simulink model "parallel_prediction_and_cost_function_6phase"  (R2022a)
settings: Solver=FixedStepDiscrete  StartTime=0.0  StopTime=10.0  RelTol=1e-3
undefined symbols (not defined in the file or in its folder): f_c, L_d, L_q, L_x, L_y, p, psi_pm, R_ph
libraries: hdlsllib x5
(part 2 of 3)

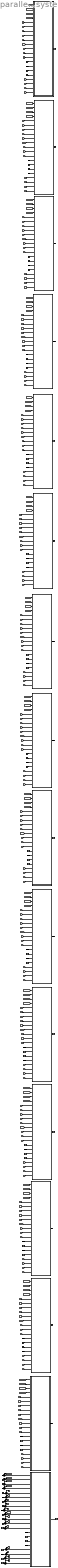
== system parallel_prediction_and_cost_function_6phase/Prediction_and_cost_function/Subsystem ==
  d_phase_voltage_per_switching_state : Inport
  q_phase_voltage_per_switching_state : Inport  Port=2
  x_phase_voltage_per_switching_state : Inport  Port=3
  y_phase_voltage_per_switching_state : Inport  Port=4
  d_phase_voltage_per_switching_state1 : Inport  Port=5
  q_phase_voltage_per_switching_state1 : Inport  Port=6
  x_phase_voltage_per_switching_state1 : Inport  Port=7
  y_phase_voltage_per_switching_state1 : Inport  Port=8
  d_phase_voltage_per_switching_state2 : Inport  Port=9
  q_phase_voltage_per_switching_state2 : Inport  Port=10
  x_phase_voltage_per_switching_state2 : Inport  Port=11
  y_phase_voltage_per_switching_state2 : Inport  Port=12
  d_phase_voltage_per_switching_state3 : Inport  Port=13
  q_phase_voltage_per_switching_state3 : Inport  Port=14
  x_phase_voltage_per_switching_state3 : Inport  Port=15
  y_phase_voltage_per_switching_state3 : Inport  Port=16
  d_phase_voltage_per_switching_state4 : Inport  Port=17
  q_phase_voltage_per_switching_state4 : Inport  Port=18
  x_phase_voltage_per_switching_state4 : Inport  Port=19
  y_phase_voltage_per_switching_state4 : Inport  Port=20
  d_phase_voltage_per_switching_state5 : Inport  Port=21
  q_phase_voltage_per_switching_state5 : Inport  Port=22
  x_phase_voltage_per_switching_state5 : Inport  Port=23
  y_phase_voltage_per_switching_state5 : Inport  Port=24
  d_phase_voltage_per_switching_state6 : Inport  Port=25
  q_phase_voltage_per_switching_state6 : Inport  Port=26
  x_phase_voltage_per_switching_state6 : Inport  Port=27
  y_phase_voltage_per_switching_state6 : Inport  Port=28
  d_phase_voltage_per_switching_state7 : Inport  Port=29
  q_phase_voltage_per_switching_state7 : Inport  Port=30
  x_phase_voltage_per_switching_state7 : Inport  Port=31
  y_phase_voltage_per_switching_state7 : Inport  Port=32
  d_phase_voltage_per_switching_state8 : Inport  Port=33
  q_phase_voltage_per_switching_state8 : Inport  Port=34
  x_phase_voltage_per_switching_state8 : Inport  Port=35
  y_phase_voltage_per_switching_state8 : Inport  Port=36
  d_phase_voltage_per_switching_state9 : Inport  Port=37
  q_phase_voltage_per_switching_state9 : Inport  Port=38
  x_phase_voltage_per_switching_state9 : Inport  Port=39
  y_phase_voltage_per_switching_state9 : Inport  Port=40
  d_phase_voltage_per_switching_state10 : Inport  Port=41
  q_phase_voltage_per_switching_state10 : Inport  Port=42
  x_phase_voltage_per_switching_state10 : Inport  Port=43
  y_phase_voltage_per_switching_state10 : Inport  Port=44
  d_phase_voltage_per_switching_state11 : Inport  Port=45
  q_phase_voltage_per_switching_state11 : Inport  Port=46
  x_phase_voltage_per_switching_state11 : Inport  Port=47
  y_phase_voltage_per_switching_state11 : Inport  Port=48
  d_phase_voltage_per_switching_state12 : Inport  Port=49
  q_phase_voltage_per_switching_state12 : Inport  Port=50
  x_phase_voltage_per_switching_state12 : Inport  Port=51
  y_phase_voltage_per_switching_state12 : Inport  Port=52
  d_phase_voltage_per_switching_state13 : Inport  Port=53
  q_phase_voltage_per_switching_state13 : Inport  Port=54
  x_phase_voltage_per_switching_state13 : Inport  Port=55
  y_phase_voltage_per_switching_state13 : Inport  Port=56
  d_phase_voltage_per_switching_state14 : Inport  Port=57
  q_phase_voltage_per_switching_state14 : Inport  Port=58
  x_phase_voltage_per_switching_state14 : Inport  Port=59
  y_phase_voltage_per_switching_state14 : Inport  Port=60
  SampleTime_div_Ld15 : Inport  Port=61
  SampleTime_div_Lq15 : Inport  Port=62
  SampleTime_div_Lx15 : Inport  Port=63
  SampleTime_div_Ly15 : Inport  Port=64
  id_k_16 : Inport  Port=65
  iq_k_16 : Inport  Port=66
  ix_k_16 : Inport  Port=67
  iy_k_16 : Inport  Port=68
  Rs15 : Inport  Port=69
  omega_el15 : Inport  Port=70
  Lq15 : Inport  Port=71
  Ld15 : Inport  Port=72
  psiPM15 : Inport  Port=73
  d_phase_voltage_per_switching_state15 : Inport  Port=74
  q_phase_voltage_per_switching_state15 : Inport  Port=75
  x_phase_voltage_per_switching_state15 : Inport  Port=76
  y_phase_voltage_per_switching_state15 : Inport  Port=77
  id_ref15 : Inport  Port=78
  iq_ref15 : Inport  Port=79
  ix_ref15 : Inport  Port=80
  iy_ref15 : Inport  Port=81
  MATLAB Function : MATLAB Function  TreatAsAtomicUnit=on
  MATLAB Function1 : MATLAB Function  TreatAsAtomicUnit=on
  MATLAB Function10 : MATLAB Function  TreatAsAtomicUnit=on
  MATLAB Function11 : MATLAB Function  TreatAsAtomicUnit=on
  MATLAB Function12 : MATLAB Function  TreatAsAtomicUnit=on
  MATLAB Function13 : MATLAB Function  TreatAsAtomicUnit=on
  MATLAB Function14 : MATLAB Function  TreatAsAtomicUnit=on
  MATLAB Function15 : MATLAB Function  TreatAsAtomicUnit=on
  MATLAB Function2 : MATLAB Function  TreatAsAtomicUnit=on
  MATLAB Function3 : MATLAB Function  TreatAsAtomicUnit=on
  MATLAB Function4 : MATLAB Function  TreatAsAtomicUnit=on
  MATLAB Function5 : MATLAB Function  TreatAsAtomicUnit=on
  MATLAB Function6 : MATLAB Function  TreatAsAtomicUnit=on
  MATLAB Function7 : MATLAB Function  TreatAsAtomicUnit=on
  MATLAB Function8 : MATLAB Function  TreatAsAtomicUnit=on
  MATLAB Function9 : MATLAB Function  TreatAsAtomicUnit=on
  J : Outport
  J1 : Outport  Port=2
  J2 : Outport  Port=3
  J3 : Outport  Port=4
  J4 : Outport  Port=5
  J5 : Outport  Port=6
  J6 : Outport  Port=7
  J7 : Outport  Port=8
  J8 : Outport  Port=9
  J9 : Outport  Port=10
  J10 : Outport  Port=11
  J11 : Outport  Port=12
  J12 : Outport  Port=13
  J13 : Outport  Port=14
  J14 : Outport  Port=15
  J15 : Outport  Port=16
  wires:
  d_phase_voltage_per_switching_state13/1 -> MATLAB Function2/14(d_phase_voltage_per_switching_state)
  q_phase_voltage_per_switching_state1/1 -> MATLAB Function14/15(q_phase_voltage_per_switching_state)
  [SampleTime_div_Ld] -> MATLAB Function15/1(SampleTime_div_Ld)
  x_phase_voltage_per_switching_state12/1 -> MATLAB Function3/16(x_phase_voltage_per_switching_state)
  [SampleTime_div_Lx] -> MATLAB Function10/3(SampleTime_div_Lx)
  SampleTime_div_Ly15/1 -> [SampleTime_div_Ly], MATLAB Function/4(SampleTime_div_Ly)
  iq_k_16/1 -> [iq_k], MATLAB Function/6(iq_k_1)
  Rs15/1 -> [Rs], MATLAB Function/9(Rs)
  iy_k_16/1 -> [iy_k], MATLAB Function/8(iy_k_1)
  MATLAB Function/1(J) -> J15/1
  y_phase_voltage_per_switching_state/1 -> MATLAB Function15/17(y_phase_voltage_per_switching_state)
  Lq15/1 -> [Lq], MATLAB Function/11(Lq)
  x_phase_voltage_per_switching_state15/1 -> MATLAB Function/16(x_phase_voltage_per_switching_state)
  MATLAB Function11/1(J) -> J4/1
  SampleTime_div_Lq15/1 -> [SampleTime_div_Lq], MATLAB Function/2(SampleTime_div_Lq)
  MATLAB Function4/1(J) -> J11/1
  y_phase_voltage_per_switching_state2/1 -> MATLAB Function13/17(y_phase_voltage_per_switching_state)
  d_phase_voltage_per_switching_state1/1 -> MATLAB Function14/14(d_phase_voltage_per_switching_state)
  iq_ref15/1 -> [iq_ref], MATLAB Function/19(iq_ref)
  SampleTime_div_Lx15/1 -> [SampleTime_div_Lx], MATLAB Function/3(SampleTime_div_Lx)
  d_phase_voltage_per_switching_state15/1 -> MATLAB Function/14(d_phase_voltage_per_switching_state)
  x_phase_voltage_per_switching_state1/1 -> MATLAB Function14/16(x_phase_voltage_per_switching_state)
  y_phase_voltage_per_switching_state7/1 -> MATLAB Function8/17(y_phase_voltage_per_switching_state)
  iy_ref15/1 -> [iy_ref], MATLAB Function/21(iy_ref)
  id_ref15/1 -> [id_ref], MATLAB Function/18(id_ref)
  id_k_16/1 -> [id_k], MATLAB Function/5(id_k_1)
  omega_el15/1 -> [omega_el], MATLAB Function/10(omega_el)
  ix_k_16/1 -> [ix_k], MATLAB Function/7(ix_k_1)
  psiPM15/1 -> [psiPM], MATLAB Function/13(psiPM)
  [iq_k] -> MATLAB Function10/6(iq_k_1)
  MATLAB Function1/1(J) -> J14/1
  ix_ref15/1 -> [ix_ref], MATLAB Function/20(ix_ref)
  d_phase_voltage_per_switching_state3/1 -> MATLAB Function12/14(d_phase_voltage_per_switching_state)
  SampleTime_div_Ld15/1 -> [SampleTime_div_Ld], MATLAB Function/1(SampleTime_div_Ld)
  d_phase_voltage_per_switching_state6/1 -> MATLAB Function9/14(d_phase_voltage_per_switching_state)
  x_phase_voltage_per_switching_state9/1 -> MATLAB Function6/16(x_phase_voltage_per_switching_state)
  d_phase_voltage_per_switching_state/1 -> MATLAB Function15/14(d_phase_voltage_per_switching_state)
  x_phase_voltage_per_switching_state3/1 -> MATLAB Function12/16(x_phase_voltage_per_switching_state)
  y_phase_voltage_per_switching_state15/1 -> MATLAB Function/17(y_phase_voltage_per_switching_state)
  d_phase_voltage_per_switching_state2/1 -> MATLAB Function13/14(d_phase_voltage_per_switching_state)
  q_phase_voltage_per_switching_state15/1 -> MATLAB Function/15(q_phase_voltage_per_switching_state)
  x_phase_voltage_per_switching_state8/1 -> MATLAB Function7/16(x_phase_voltage_per_switching_state)
  y_phase_voltage_per_switching_state9/1 -> MATLAB Function6/17(y_phase_voltage_per_switching_state)
  x_phase_voltage_per_switching_state4/1 -> MATLAB Function11/16(x_phase_voltage_per_switching_state)
  y_phase_voltage_per_switching_state1/1 -> MATLAB Function14/17(y_phase_voltage_per_switching_state)
  MATLAB Function14/1(J) -> J1/1
  MATLAB Function8/1(J) -> J7/1
  [ix_ref] -> MATLAB Function2/20(ix_ref)
  q_phase_voltage_per_switching_state2/1 -> MATLAB Function13/15(q_phase_voltage_per_switching_state)
  x_phase_voltage_per_switching_state2/1 -> MATLAB Function13/16(x_phase_voltage_per_switching_state)
  [iq_ref] -> MATLAB Function9/19(iq_ref)
  MATLAB Function13/1(J) -> J2/1
  y_phase_voltage_per_switching_state11/1 -> MATLAB Function4/17(y_phase_voltage_per_switching_state)
  [SampleTime_div_Ly] -> MATLAB Function10/4(SampleTime_div_Ly)
  y_phase_voltage_per_switching_state4/1 -> MATLAB Function11/17(y_phase_voltage_per_switching_state)
  x_phase_voltage_per_switching_state/1 -> MATLAB Function15/16(x_phase_voltage_per_switching_state)
  d_phase_voltage_per_switching_state14/1 -> MATLAB Function1/14(d_phase_voltage_per_switching_state)
  q_phase_voltage_per_switching_state9/1 -> MATLAB Function6/15(q_phase_voltage_per_switching_state)
  q_phase_voltage_per_switching_state5/1 -> MATLAB Function10/15(q_phase_voltage_per_switching_state)
  d_phase_voltage_per_switching_state10/1 -> MATLAB Function5/14(d_phase_voltage_per_switching_state)
  x_phase_voltage_per_switching_state14/1 -> MATLAB Function1/16(x_phase_voltage_per_switching_state)
  y_phase_voltage_per_switching_state14/1 -> MATLAB Function1/17(y_phase_voltage_per_switching_state)
  q_phase_voltage_per_switching_state14/1 -> MATLAB Function1/15(q_phase_voltage_per_switching_state)
  [iy_k] -> MATLAB Function10/8(iy_k_1)
  q_phase_voltage_per_switching_state11/1 -> MATLAB Function4/15(q_phase_voltage_per_switching_state)
  x_phase_voltage_per_switching_state11/1 -> MATLAB Function4/16(x_phase_voltage_per_switching_state)
  d_phase_voltage_per_switching_state11/1 -> MATLAB Function4/14(d_phase_voltage_per_switching_state)
  MATLAB Function2/1(J) -> J13/1
  y_phase_voltage_per_switching_state12/1 -> MATLAB Function3/17(y_phase_voltage_per_switching_state)
  x_phase_voltage_per_switching_state13/1 -> MATLAB Function2/16(x_phase_voltage_per_switching_state)
  [SampleTime_div_Ld] -> MATLAB Function12/1(SampleTime_div_Ld)
  [id_ref] -> MATLAB Function2/18(id_ref)
  d_phase_voltage_per_switching_state9/1 -> MATLAB Function6/14(d_phase_voltage_per_switching_state)
  MATLAB Function6/1(J) -> J9/1
  d_phase_voltage_per_switching_state7/1 -> MATLAB Function8/14(d_phase_voltage_per_switching_state)
  d_phase_voltage_per_switching_state4/1 -> MATLAB Function11/14(d_phase_voltage_per_switching_state)
  q_phase_voltage_per_switching_state4/1 -> MATLAB Function11/15(q_phase_voltage_per_switching_state)
  q_phase_voltage_per_switching_state12/1 -> MATLAB Function3/15(q_phase_voltage_per_switching_state)
  [iy_ref] -> MATLAB Function2/21(iy_ref)
  d_phase_voltage_per_switching_state8/1 -> MATLAB Function7/14(d_phase_voltage_per_switching_state)
  x_phase_voltage_per_switching_state5/1 -> MATLAB Function10/16(x_phase_voltage_per_switching_state)
  d_phase_voltage_per_switching_state12/1 -> MATLAB Function3/14(d_phase_voltage_per_switching_state)
  MATLAB Function3/1(J) -> J12/1
  [SampleTime_div_Lx] -> MATLAB Function15/3(SampleTime_div_Lx)
  [SampleTime_div_Ly] -> MATLAB Function15/4(SampleTime_div_Ly)
  [SampleTime_div_Lq] -> MATLAB Function15/2(SampleTime_div_Lq)
  [SampleTime_div_Ld] -> MATLAB Function10/1(SampleTime_div_Ld)
  [SampleTime_div_Lx] -> MATLAB Function12/3(SampleTime_div_Lx)
  [SampleTime_div_Lq] -> MATLAB Function10/2(SampleTime_div_Lq)
  x_phase_voltage_per_switching_state7/1 -> MATLAB Function8/16(x_phase_voltage_per_switching_state)
  q_phase_voltage_per_switching_state/1 -> MATLAB Function15/15(q_phase_voltage_per_switching_state)
  [SampleTime_div_Lq] -> MATLAB Function12/2(SampleTime_div_Lq)
  MATLAB Function15/1(J) -> J/1
  [id_k] -> MATLAB Function10/5(id_k_1)
  [ix_k] -> MATLAB Function10/7(ix_k_1)
  d_phase_voltage_per_switching_state5/1 -> MATLAB Function10/14(d_phase_voltage_per_switching_state)
  q_phase_voltage_per_switching_state13/1 -> MATLAB Function2/15(q_phase_voltage_per_switching_state)
  MATLAB Function10/1(J) -> J5/1
  y_phase_voltage_per_switching_state5/1 -> MATLAB Function10/17(y_phase_voltage_per_switching_state)
  MATLAB Function5/1(J) -> J10/1
  q_phase_voltage_per_switching_state6/1 -> MATLAB Function9/15(q_phase_voltage_per_switching_state)
  y_phase_voltage_per_switching_state6/1 -> MATLAB Function9/17(y_phase_voltage_per_switching_state)
  [ix_ref] -> MATLAB Function9/20(ix_ref)
  [id_ref] -> MATLAB Function9/18(id_ref)
  x_phase_voltage_per_switching_state6/1 -> MATLAB Function9/16(x_phase_voltage_per_switching_state)
  MATLAB Function9/1(J) -> J6/1
  [iy_ref] -> MATLAB Function9/21(iy_ref)
  y_phase_voltage_per_switching_state8/1 -> MATLAB Function7/17(y_phase_voltage_per_switching_state)
  MATLAB Function12/1(J) -> J3/1
  q_phase_voltage_per_switching_state8/1 -> MATLAB Function7/15(q_phase_voltage_per_switching_state)
  y_phase_voltage_per_switching_state13/1 -> MATLAB Function2/17(y_phase_voltage_per_switching_state)
  MATLAB Function7/1(J) -> J8/1
  q_phase_voltage_per_switching_state7/1 -> MATLAB Function8/15(q_phase_voltage_per_switching_state)
  [iq_ref] -> MATLAB Function2/19(iq_ref)
  [SampleTime_div_Ly] -> MATLAB Function12/4(SampleTime_div_Ly)
  x_phase_voltage_per_switching_state10/1 -> MATLAB Function5/16(x_phase_voltage_per_switching_state)
  q_phase_voltage_per_switching_state10/1 -> MATLAB Function5/15(q_phase_voltage_per_switching_state)
  y_phase_voltage_per_switching_state10/1 -> MATLAB Function5/17(y_phase_voltage_per_switching_state)
  y_phase_voltage_per_switching_state3/1 -> MATLAB Function12/17(y_phase_voltage_per_switching_state)
  q_phase_voltage_per_switching_state3/1 -> MATLAB Function12/15(q_phase_voltage_per_switching_state)
  [SampleTime_div_Ld] -> MATLAB Function1/1(SampleTime_div_Ld)
  [SampleTime_div_Ld] -> MATLAB Function2/1(SampleTime_div_Ld)
  [SampleTime_div_Ld] -> MATLAB Function3/1(SampleTime_div_Ld)
  [SampleTime_div_Ld] -> MATLAB Function4/1(SampleTime_div_Ld)
  [SampleTime_div_Ld] -> MATLAB Function6/1(SampleTime_div_Ld)
  [SampleTime_div_Ld] -> MATLAB Function5/1(SampleTime_div_Ld)
  [SampleTime_div_Ld] -> MATLAB Function7/1(SampleTime_div_Ld)
  [SampleTime_div_Ld] -> MATLAB Function8/1(SampleTime_div_Ld)
  [SampleTime_div_Ld] -> MATLAB Function9/1(SampleTime_div_Ld)
  [SampleTime_div_Ld] -> MATLAB Function11/1(SampleTime_div_Ld)
  [SampleTime_div_Ld] -> MATLAB Function13/1(SampleTime_div_Ld)
  [SampleTime_div_Ld] -> MATLAB Function14/1(SampleTime_div_Ld)
  [SampleTime_div_Lq] -> MATLAB Function1/2(SampleTime_div_Lq)
  [SampleTime_div_Lq] -> MATLAB Function2/2(SampleTime_div_Lq)
  [SampleTime_div_Lq] -> MATLAB Function3/2(SampleTime_div_Lq)
  [SampleTime_div_Lq] -> MATLAB Function4/2(SampleTime_div_Lq)
  [SampleTime_div_Lq] -> MATLAB Function5/2(SampleTime_div_Lq)
  [SampleTime_div_Lq] -> MATLAB Function6/2(SampleTime_div_Lq)
  [SampleTime_div_Lq] -> MATLAB Function7/2(SampleTime_div_Lq)
  [SampleTime_div_Lq] -> MATLAB Function8/2(SampleTime_div_Lq)
  [SampleTime_div_Lq] -> MATLAB Function9/2(SampleTime_div_Lq)
  [SampleTime_div_Lq] -> MATLAB Function11/2(SampleTime_div_Lq)
  [SampleTime_div_Lq] -> MATLAB Function13/2(SampleTime_div_Lq)
  [SampleTime_div_Lq] -> MATLAB Function14/2(SampleTime_div_Lq)
  [SampleTime_div_Lx] -> MATLAB Function1/3(SampleTime_div_Lx)
  [SampleTime_div_Lx] -> MATLAB Function2/3(SampleTime_div_Lx)
  [SampleTime_div_Lx] -> MATLAB Function3/3(SampleTime_div_Lx)
  [SampleTime_div_Lx] -> MATLAB Function4/3(SampleTime_div_Lx)
  [SampleTime_div_Lx] -> MATLAB Function5/3(SampleTime_div_Lx)
  [SampleTime_div_Lx] -> MATLAB Function6/3(SampleTime_div_Lx)
  [SampleTime_div_Lx] -> MATLAB Function7/3(SampleTime_div_Lx)
  [SampleTime_div_Lx] -> MATLAB Function8/3(SampleTime_div_Lx)
  [SampleTime_div_Lx] -> MATLAB Function9/3(SampleTime_div_Lx)
  [SampleTime_div_Lx] -> MATLAB Function11/3(SampleTime_div_Lx)
  [SampleTime_div_Lx] -> MATLAB Function13/3(SampleTime_div_Lx)
  [SampleTime_div_Lx] -> MATLAB Function14/3(SampleTime_div_Lx)
  [SampleTime_div_Ly] -> MATLAB Function1/4(SampleTime_div_Ly)
  [SampleTime_div_Ly] -> MATLAB Function2/4(SampleTime_div_Ly)
  [SampleTime_div_Ly] -> MATLAB Function3/4(SampleTime_div_Ly)
  [SampleTime_div_Ly] -> MATLAB Function4/4(SampleTime_div_Ly)
  [SampleTime_div_Ly] -> MATLAB Function5/4(SampleTime_div_Ly)
  [SampleTime_div_Ly] -> MATLAB Function6/4(SampleTime_div_Ly)
  [SampleTime_div_Ly] -> MATLAB Function7/4(SampleTime_div_Ly)
  [SampleTime_div_Ly] -> MATLAB Function8/4(SampleTime_div_Ly)
  [SampleTime_div_Ly] -> MATLAB Function9/4(SampleTime_div_Ly)
  [SampleTime_div_Ly] -> MATLAB Function11/4(SampleTime_div_Ly)
  [SampleTime_div_Ly] -> MATLAB Function13/4(SampleTime_div_Ly)
  [SampleTime_div_Ly] -> MATLAB Function14/4(SampleTime_div_Ly)
  [id_k] -> MATLAB Function1/5(id_k_1)
  [iq_k] -> MATLAB Function1/6(iq_k_1)
  [ix_k] -> MATLAB Function1/7(ix_k_1)
  [iy_k] -> MATLAB Function1/8(iy_k_1)
  [Rs] -> MATLAB Function1/9(Rs)
  [omega_el] -> MATLAB Function1/10(omega_el)
  [Lq] -> MATLAB Function1/11(Lq)
  Ld15/1 -> [Ld], MATLAB Function/12(Ld)
  [Ld] -> MATLAB Function1/12(Ld)
  [psiPM] -> MATLAB Function1/13(psiPM)
  [id_ref] -> MATLAB Function1/18(id_ref)
  [iq_ref] -> MATLAB Function1/19(iq_ref)
  [ix_ref] -> MATLAB Function1/20(ix_ref)
  [iy_ref] -> MATLAB Function1/21(iy_ref)
  [Ld] -> MATLAB Function2/12(Ld)
  [omega_el] -> MATLAB Function2/10(omega_el)
  [iy_k] -> MATLAB Function2/8(iy_k_1)
  [Lq] -> MATLAB Function2/11(Lq)
  [psiPM] -> MATLAB Function2/13(psiPM)
  [iq_k] -> MATLAB Function2/6(iq_k_1)
  [id_k] -> MATLAB Function2/5(id_k_1)
  [ix_k] -> MATLAB Function2/7(ix_k_1)
  [Rs] -> MATLAB Function2/9(Rs)
  [Ld] -> MATLAB Function3/12(Ld)
  [omega_el] -> MATLAB Function3/10(omega_el)
  [iy_k] -> MATLAB Function3/8(iy_k_1)
  [Lq] -> MATLAB Function3/11(Lq)
  [psiPM] -> MATLAB Function3/13(psiPM)
  [iq_ref] -> MATLAB Function3/19(iq_ref)
  [iq_k] -> MATLAB Function3/6(iq_k_1)
  [id_k] -> MATLAB Function3/5(id_k_1)
  [iy_ref] -> MATLAB Function3/21(iy_ref)
  [ix_k] -> MATLAB Function3/7(ix_k_1)
  [Rs] -> MATLAB Function3/9(Rs)
  [id_ref] -> MATLAB Function3/18(id_ref)
  [ix_ref] -> MATLAB Function3/20(ix_ref)
  [Ld] -> MATLAB Function4/12(Ld)
  [omega_el] -> MATLAB Function4/10(omega_el)
  [iy_k] -> MATLAB Function4/8(iy_k_1)
  [Lq] -> MATLAB Function4/11(Lq)
  [psiPM] -> MATLAB Function4/13(psiPM)
  [iq_ref] -> MATLAB Function4/19(iq_ref)
  [iq_k] -> MATLAB Function4/6(iq_k_1)
  [id_k] -> MATLAB Function4/5(id_k_1)
  [iy_ref] -> MATLAB Function4/21(iy_ref)
  [ix_k] -> MATLAB Function4/7(ix_k_1)
  [Rs] -> MATLAB Function4/9(Rs)
  [id_ref] -> MATLAB Function4/18(id_ref)
  [ix_ref] -> MATLAB Function4/20(ix_ref)
  [Ld] -> MATLAB Function5/12(Ld)
  [omega_el] -> MATLAB Function5/10(omega_el)
  [iy_k] -> MATLAB Function5/8(iy_k_1)
  [Lq] -> MATLAB Function5/11(Lq)
  [psiPM] -> MATLAB Function5/13(psiPM)
  [iq_ref] -> MATLAB Function5/19(iq_ref)
  [iq_k] -> MATLAB Function5/6(iq_k_1)
  [id_k] -> MATLAB Function5/5(id_k_1)
  [iy_ref] -> MATLAB Function5/21(iy_ref)
  [ix_k] -> MATLAB Function5/7(ix_k_1)
  [Rs] -> MATLAB Function5/9(Rs)
  [id_ref] -> MATLAB Function5/18(id_ref)
  [ix_ref] -> MATLAB Function5/20(ix_ref)
  [Ld] -> MATLAB Function6/12(Ld)
  [omega_el] -> MATLAB Function6/10(omega_el)
  [iy_k] -> MATLAB Function6/8(iy_k_1)
  [Lq] -> MATLAB Function6/11(Lq)
  [psiPM] -> MATLAB Function6/13(psiPM)
  [iq_ref] -> MATLAB Function6/19(iq_ref)
  [iq_k] -> MATLAB Function6/6(iq_k_1)
  [id_k] -> MATLAB Function6/5(id_k_1)
  [iy_ref] -> MATLAB Function6/21(iy_ref)
  [ix_k] -> MATLAB Function6/7(ix_k_1)
  [Rs] -> MATLAB Function6/9(Rs)
  [id_ref] -> MATLAB Function6/18(id_ref)
  [ix_ref] -> MATLAB Function6/20(ix_ref)
  [Ld] -> MATLAB Function7/12(Ld)
  [omega_el] -> MATLAB Function7/10(omega_el)
  [iy_k] -> MATLAB Function7/8(iy_k_1)
  [Lq] -> MATLAB Function7/11(Lq)
  [psiPM] -> MATLAB Function7/13(psiPM)
  [iq_ref] -> MATLAB Function7/19(iq_ref)
  [iq_k] -> MATLAB Function7/6(iq_k_1)
  [id_k] -> MATLAB Function7/5(id_k_1)
  [iy_ref] -> MATLAB Function7/21(iy_ref)
  [ix_k] -> MATLAB Function7/7(ix_k_1)
  [Rs] -> MATLAB Function7/9(Rs)
  [id_ref] -> MATLAB Function7/18(id_ref)
  [ix_ref] -> MATLAB Function7/20(ix_ref)
  [Ld] -> MATLAB Function8/12(Ld)
  [omega_el] -> MATLAB Function8/10(omega_el)
  [iy_k] -> MATLAB Function8/8(iy_k_1)
  [Lq] -> MATLAB Function8/11(Lq)
  [psiPM] -> MATLAB Function8/13(psiPM)
  [iq_ref] -> MATLAB Function8/19(iq_ref)
  [iq_k] -> MATLAB Function8/6(iq_k_1)
  [id_k] -> MATLAB Function8/5(id_k_1)
  [iy_ref] -> MATLAB Function8/21(iy_ref)
  [ix_k] -> MATLAB Function8/7(ix_k_1)
  [Rs] -> MATLAB Function8/9(Rs)
  [id_ref] -> MATLAB Function8/18(id_ref)
  [ix_ref] -> MATLAB Function8/20(ix_ref)
  [Ld] -> MATLAB Function9/12(Ld)
  [omega_el] -> MATLAB Function9/10(omega_el)
  [iy_k] -> MATLAB Function9/8(iy_k_1)
  [Lq] -> MATLAB Function9/11(Lq)
  [psiPM] -> MATLAB Function9/13(psiPM)
  [iq_k] -> MATLAB Function9/6(iq_k_1)
  [id_k] -> MATLAB Function9/5(id_k_1)
  [ix_k] -> MATLAB Function9/7(ix_k_1)
  [Rs] -> MATLAB Function9/9(Rs)
  [Ld] -> MATLAB Function10/12(Ld)
  [Lq] -> MATLAB Function10/11(Lq)
  [psiPM] -> MATLAB Function10/13(psiPM)
  [iq_ref] -> MATLAB Function10/19(iq_ref)
  [iy_ref] -> MATLAB Function10/21(iy_ref)
  [id_ref] -> MATLAB Function10/18(id_ref)
  [ix_ref] -> MATLAB Function10/20(ix_ref)
  [Rs] -> MATLAB Function10/9(Rs)
  [omega_el] -> MATLAB Function10/10(omega_el)
  [Ld] -> MATLAB Function11/12(Ld)
  [omega_el] -> MATLAB Function11/10(omega_el)
  [iy_k] -> MATLAB Function11/8(iy_k_1)
  [Lq] -> MATLAB Function11/11(Lq)
  [psiPM] -> MATLAB Function11/13(psiPM)
  [iq_ref] -> MATLAB Function11/19(iq_ref)
  [iq_k] -> MATLAB Function11/6(iq_k_1)
  [id_k] -> MATLAB Function11/5(id_k_1)
  [iy_ref] -> MATLAB Function11/21(iy_ref)
  [ix_k] -> MATLAB Function11/7(ix_k_1)
  [Rs] -> MATLAB Function11/9(Rs)
  [id_ref] -> MATLAB Function11/18(id_ref)
  [ix_ref] -> MATLAB Function11/20(ix_ref)
  [Ld] -> MATLAB Function12/12(Ld)
  [omega_el] -> MATLAB Function12/10(omega_el)
  [iy_k] -> MATLAB Function12/8(iy_k_1)
  [Lq] -> MATLAB Function12/11(Lq)
  [psiPM] -> MATLAB Function12/13(psiPM)
  [iq_ref] -> MATLAB Function12/19(iq_ref)
  [iq_k] -> MATLAB Function12/6(iq_k_1)
  [id_k] -> MATLAB Function12/5(id_k_1)
  [iy_ref] -> MATLAB Function12/21(iy_ref)
  [ix_k] -> MATLAB Function12/7(ix_k_1)
  [Rs] -> MATLAB Function12/9(Rs)
  [id_ref] -> MATLAB Function12/18(id_ref)
  [ix_ref] -> MATLAB Function12/20(ix_ref)
  [Ld] -> MATLAB Function13/12(Ld)
  [omega_el] -> MATLAB Function13/10(omega_el)
  [iy_k] -> MATLAB Function13/8(iy_k_1)
  [Lq] -> MATLAB Function13/11(Lq)
  [psiPM] -> MATLAB Function13/13(psiPM)
  [iq_ref] -> MATLAB Function13/19(iq_ref)
  [iq_k] -> MATLAB Function13/6(iq_k_1)
  [id_k] -> MATLAB Function13/5(id_k_1)
  [iy_ref] -> MATLAB Function13/21(iy_ref)
  [ix_k] -> MATLAB Function13/7(ix_k_1)
  [Rs] -> MATLAB Function13/9(Rs)
  [id_ref] -> MATLAB Function13/18(id_ref)
  [ix_ref] -> MATLAB Function13/20(ix_ref)
  [Ld] -> MATLAB Function14/12(Ld)
  [omega_el] -> MATLAB Function14/10(omega_el)
  [iy_k] -> MATLAB Function14/8(iy_k_1)
  [Lq] -> MATLAB Function14/11(Lq)
  [psiPM] -> MATLAB Function14/13(psiPM)
  [iq_ref] -> MATLAB Function14/19(iq_ref)
  [iq_k] -> MATLAB Function14/6(iq_k_1)
  [id_k] -> MATLAB Function14/5(id_k_1)
  [iy_ref] -> MATLAB Function14/21(iy_ref)
  [ix_k] -> MATLAB Function14/7(ix_k_1)
  [Rs] -> MATLAB Function14/9(Rs)
  [id_ref] -> MATLAB Function14/18(id_ref)
  [ix_ref] -> MATLAB Function14/20(ix_ref)
  [Ld] -> MATLAB Function15/12(Ld)
  [omega_el] -> MATLAB Function15/10(omega_el)
  [iy_k] -> MATLAB Function15/8(iy_k_1)
  [Lq] -> MATLAB Function15/11(Lq)
  [psiPM] -> MATLAB Function15/13(psiPM)
  [iq_ref] -> MATLAB Function15/19(iq_ref)
  [iq_k] -> MATLAB Function15/6(iq_k_1)
  [id_k] -> MATLAB Function15/5(id_k_1)
  [iy_ref] -> MATLAB Function15/21(iy_ref)
  [ix_k] -> MATLAB Function15/7(ix_k_1)
  [Rs] -> MATLAB Function15/9(Rs)
  [id_ref] -> MATLAB Function15/18(id_ref)
  [ix_ref] -> MATLAB Function15/20(ix_ref)

== matlab function parallel_prediction_and_cost_function_6phase/Prediction_and_cost_function/Subsystem/MATLAB Function3 ==
  data: SampleTime_div_Ld input; J output; SampleTime_div_Lq input; SampleTime_div_Lx input; SampleTime_div_Ly input; id_k_1 input; iq_k_1 input; ix_k_1 input; iy_k_1 input; Rs input; omega_el input; Lq input; Ld input; psiPM input; d_phase_voltage_per_switching_state input; q_phase_voltage_per_switching_state input; x_phase_voltage_per_switching_state input; y_phase_voltage_per_switching_state input; id_ref input; iq_ref input; ix_ref input; iy_ref input
function J = fcn(SampleTime_div_Ld, SampleTime_div_Lq, SampleTime_div_Lx, SampleTime_div_Ly, id_k_1, iq_k_1, ix_k_1, iy_k_1, Rs, omega_el, Lq, Ld, psiPM, d_phase_voltage_per_switching_state, q_phase_voltage_per_switching_state, x_phase_voltage_per_switching_state, y_phase_voltage_per_switching_state, id_ref, iq_ref, ix_ref, iy_ref)
     
        % Prediction of the d-, q-, x-, y-currents of the 6-Phase-PMSM with the finite control set 
        id_k_2 = single(SampleTime_div_Ld*(d_phase_voltage_per_switching_state-id_k_1*Rs+omega_el*Lq*iq_k_1)+id_k_1);
        iq_k_2 = single(SampleTime_div_Lq*(q_phase_voltage_per_switching_state-iq_k_1*Rs-omega_el*(psiPM+id_k_1*Ld))+iq_k_1);
        ix_k_2 = single(SampleTime_div_Lx*(x_phase_voltage_per_switching_state-ix_k_1*Rs)+ix_k_1);
        iy_k_2 = single(SampleTime_div_Ly*(y_phase_voltage_per_switching_state-iy_k_1*Rs)+iy_k_1);
        
        % Calculation of the cost function
        J = single((id_ref-id_k_2)^2+(iq_ref-iq_k_2)^2+(ix_ref-ix_k_2)^2+(iy_ref-iy_k_2)^2);

end

== matlab function parallel_prediction_and_cost_function_6phase/Prediction_and_cost_function/Subsystem/MATLAB Function4 ==
  data: SampleTime_div_Ld input; J output; SampleTime_div_Lq input; SampleTime_div_Lx input; SampleTime_div_Ly input; id_k_1 input; iq_k_1 input; ix_k_1 input; iy_k_1 input; Rs input; omega_el input; Lq input; Ld input; psiPM input; d_phase_voltage_per_switching_state input; q_phase_voltage_per_switching_state input; x_phase_voltage_per_switching_state input; y_phase_voltage_per_switching_state input; id_ref input; iq_ref input; ix_ref input; iy_ref input
function J = fcn(SampleTime_div_Ld, SampleTime_div_Lq, SampleTime_div_Lx, SampleTime_div_Ly, id_k_1, iq_k_1, ix_k_1, iy_k_1, Rs, omega_el, Lq, Ld, psiPM, d_phase_voltage_per_switching_state, q_phase_voltage_per_switching_state, x_phase_voltage_per_switching_state, y_phase_voltage_per_switching_state, id_ref, iq_ref, ix_ref, iy_ref)
     
        % Prediction of the d-, q-, x-, y-currents of the 6-Phase-PMSM with the finite control set 
        id_k_2 = single(SampleTime_div_Ld*(d_phase_voltage_per_switching_state-id_k_1*Rs+omega_el*Lq*iq_k_1)+id_k_1);
        iq_k_2 = single(SampleTime_div_Lq*(q_phase_voltage_per_switching_state-iq_k_1*Rs-omega_el*(psiPM+id_k_1*Ld))+iq_k_1);
        ix_k_2 = single(SampleTime_div_Lx*(x_phase_voltage_per_switching_state-ix_k_1*Rs)+ix_k_1);
        iy_k_2 = single(SampleTime_div_Ly*(y_phase_voltage_per_switching_state-iy_k_1*Rs)+iy_k_1);
        
        % Calculation of the cost function
        J = single((id_ref-id_k_2)^2+(iq_ref-iq_k_2)^2+(ix_ref-ix_k_2)^2+(iy_ref-iy_k_2)^2);

end

== matlab function parallel_prediction_and_cost_function_6phase/Prediction_and_cost_function/Subsystem/MATLAB Function5 ==
  data: SampleTime_div_Ld input; J output; SampleTime_div_Lq input; SampleTime_div_Lx input; SampleTime_div_Ly input; id_k_1 input; iq_k_1 input; ix_k_1 input; iy_k_1 input; Rs input; omega_el input; Lq input; Ld input; psiPM input; d_phase_voltage_per_switching_state input; q_phase_voltage_per_switching_state input; x_phase_voltage_per_switching_state input; y_phase_voltage_per_switching_state input; id_ref input; iq_ref input; ix_ref input; iy_ref input
function J = fcn(SampleTime_div_Ld, SampleTime_div_Lq, SampleTime_div_Lx, SampleTime_div_Ly, id_k_1, iq_k_1, ix_k_1, iy_k_1, Rs, omega_el, Lq, Ld, psiPM, d_phase_voltage_per_switching_state, q_phase_voltage_per_switching_state, x_phase_voltage_per_switching_state, y_phase_voltage_per_switching_state, id_ref, iq_ref, ix_ref, iy_ref)
     
        % Prediction of the d-, q-, x-, y-currents of the 6-Phase-PMSM with the finite control set 
        id_k_2 = single(SampleTime_div_Ld*(d_phase_voltage_per_switching_state-id_k_1*Rs+omega_el*Lq*iq_k_1)+id_k_1);
        iq_k_2 = single(SampleTime_div_Lq*(q_phase_voltage_per_switching_state-iq_k_1*Rs-omega_el*(psiPM+id_k_1*Ld))+iq_k_1);
        ix_k_2 = single(SampleTime_div_Lx*(x_phase_voltage_per_switching_state-ix_k_1*Rs)+ix_k_1);
        iy_k_2 = single(SampleTime_div_Ly*(y_phase_voltage_per_switching_state-iy_k_1*Rs)+iy_k_1);
        
        % Calculation of the cost function
        J = single((id_ref-id_k_2)^2+(iq_ref-iq_k_2)^2+(ix_ref-ix_k_2)^2+(iy_ref-iy_k_2)^2);

end

== matlab function parallel_prediction_and_cost_function_6phase/Prediction_and_cost_function/Subsystem/MATLAB Function6 ==
  data: SampleTime_div_Ld input; J output; SampleTime_div_Lq input; SampleTime_div_Lx input; SampleTime_div_Ly input; id_k_1 input; iq_k_1 input; ix_k_1 input; iy_k_1 input; Rs input; omega_el input; Lq input; Ld input; psiPM input; d_phase_voltage_per_switching_state input; q_phase_voltage_per_switching_state input; x_phase_voltage_per_switching_state input; y_phase_voltage_per_switching_state input; id_ref input; iq_ref input; ix_ref input; iy_ref input
function J = fcn(SampleTime_div_Ld, SampleTime_div_Lq, SampleTime_div_Lx, SampleTime_div_Ly, id_k_1, iq_k_1, ix_k_1, iy_k_1, Rs, omega_el, Lq, Ld, psiPM, d_phase_voltage_per_switching_state, q_phase_voltage_per_switching_state, x_phase_voltage_per_switching_state, y_phase_voltage_per_switching_state, id_ref, iq_ref, ix_ref, iy_ref)
     
        % Prediction of the d-, q-, x-, y-currents of the 6-Phase-PMSM with the finite control set 
        id_k_2 = single(SampleTime_div_Ld*(d_phase_voltage_per_switching_state-id_k_1*Rs+omega_el*Lq*iq_k_1)+id_k_1);
        iq_k_2 = single(SampleTime_div_Lq*(q_phase_voltage_per_switching_state-iq_k_1*Rs-omega_el*(psiPM+id_k_1*Ld))+iq_k_1);
        ix_k_2 = single(SampleTime_div_Lx*(x_phase_voltage_per_switching_state-ix_k_1*Rs)+ix_k_1);
        iy_k_2 = single(SampleTime_div_Ly*(y_phase_voltage_per_switching_state-iy_k_1*Rs)+iy_k_1);
        
        % Calculation of the cost function
        J = single((id_ref-id_k_2)^2+(iq_ref-iq_k_2)^2+(ix_ref-ix_k_2)^2+(iy_ref-iy_k_2)^2);

end

== matlab function parallel_prediction_and_cost_function_6phase/Prediction_and_cost_function/Subsystem/MATLAB Function7 ==
  data: SampleTime_div_Ld input; J output; SampleTime_div_Lq input; SampleTime_div_Lx input; SampleTime_div_Ly input; id_k_1 input; iq_k_1 input; ix_k_1 input; iy_k_1 input; Rs input; omega_el input; Lq input; Ld input; psiPM input; d_phase_voltage_per_switching_state input; q_phase_voltage_per_switching_state input; x_phase_voltage_per_switching_state input; y_phase_voltage_per_switching_state input; id_ref input; iq_ref input; ix_ref input; iy_ref input
function J = fcn(SampleTime_div_Ld, SampleTime_div_Lq, SampleTime_div_Lx, SampleTime_div_Ly, id_k_1, iq_k_1, ix_k_1, iy_k_1, Rs, omega_el, Lq, Ld, psiPM, d_phase_voltage_per_switching_state, q_phase_voltage_per_switching_state, x_phase_voltage_per_switching_state, y_phase_voltage_per_switching_state, id_ref, iq_ref, ix_ref, iy_ref)
     
        % Prediction of the d-, q-, x-, y-currents of the 6-Phase-PMSM with the finite control set 
        id_k_2 = single(SampleTime_div_Ld*(d_phase_voltage_per_switching_state-id_k_1*Rs+omega_el*Lq*iq_k_1)+id_k_1);
        iq_k_2 = single(SampleTime_div_Lq*(q_phase_voltage_per_switching_state-iq_k_1*Rs-omega_el*(psiPM+id_k_1*Ld))+iq_k_1);
        ix_k_2 = single(SampleTime_div_Lx*(x_phase_voltage_per_switching_state-ix_k_1*Rs)+ix_k_1);
        iy_k_2 = single(SampleTime_div_Ly*(y_phase_voltage_per_switching_state-iy_k_1*Rs)+iy_k_1);
        
        % Calculation of the cost function
        J = single((id_ref-id_k_2)^2+(iq_ref-iq_k_2)^2+(ix_ref-ix_k_2)^2+(iy_ref-iy_k_2)^2);

end

== matlab function parallel_prediction_and_cost_function_6phase/Prediction_and_cost_function/Subsystem/MATLAB Function8 ==
  data: SampleTime_div_Ld input; J output; SampleTime_div_Lq input; SampleTime_div_Lx input; SampleTime_div_Ly input; id_k_1 input; iq_k_1 input; ix_k_1 input; iy_k_1 input; Rs input; omega_el input; Lq input; Ld input; psiPM input; d_phase_voltage_per_switching_state input; q_phase_voltage_per_switching_state input; x_phase_voltage_per_switching_state input; y_phase_voltage_per_switching_state input; id_ref input; iq_ref input; ix_ref input; iy_ref input
function J = fcn(SampleTime_div_Ld, SampleTime_div_Lq, SampleTime_div_Lx, SampleTime_div_Ly, id_k_1, iq_k_1, ix_k_1, iy_k_1, Rs, omega_el, Lq, Ld, psiPM, d_phase_voltage_per_switching_state, q_phase_voltage_per_switching_state, x_phase_voltage_per_switching_state, y_phase_voltage_per_switching_state, id_ref, iq_ref, ix_ref, iy_ref)
     
        % Prediction of the d-, q-, x-, y-currents of the 6-Phase-PMSM with the finite control set 
        id_k_2 = single(SampleTime_div_Ld*(d_phase_voltage_per_switching_state-id_k_1*Rs+omega_el*Lq*iq_k_1)+id_k_1);
        iq_k_2 = single(SampleTime_div_Lq*(q_phase_voltage_per_switching_state-iq_k_1*Rs-omega_el*(psiPM+id_k_1*Ld))+iq_k_1);
        ix_k_2 = single(SampleTime_div_Lx*(x_phase_voltage_per_switching_state-ix_k_1*Rs)+ix_k_1);
        iy_k_2 = single(SampleTime_div_Ly*(y_phase_voltage_per_switching_state-iy_k_1*Rs)+iy_k_1);
        
        % Calculation of the cost function
        J = single((id_ref-id_k_2)^2+(iq_ref-iq_k_2)^2+(ix_ref-ix_k_2)^2+(iy_ref-iy_k_2)^2);

end

== matlab function parallel_prediction_and_cost_function_6phase/Prediction_and_cost_function/Subsystem/MATLAB Function ==
  data: SampleTime_div_Ld input; J output; SampleTime_div_Lq input; SampleTime_div_Lx input; SampleTime_div_Ly input; id_k_1 input; iq_k_1 input; ix_k_1 input; iy_k_1 input; Rs input; omega_el input; Lq input; Ld input; psiPM input; d_phase_voltage_per_switching_state input; q_phase_voltage_per_switching_state input; x_phase_voltage_per_switching_state input; y_phase_voltage_per_switching_state input; id_ref input; iq_ref input; ix_ref input; iy_ref input
function J = fcn(SampleTime_div_Ld, SampleTime_div_Lq, SampleTime_div_Lx, SampleTime_div_Ly, id_k_1, iq_k_1, ix_k_1, iy_k_1, Rs, omega_el, Lq, Ld, psiPM, d_phase_voltage_per_switching_state, q_phase_voltage_per_switching_state, x_phase_voltage_per_switching_state, y_phase_voltage_per_switching_state, id_ref, iq_ref, ix_ref, iy_ref)
     
        % Prediction of the d-, q-, x-, y-currents of the 6-Phase-PMSM with the finite control set 
        id_k_2 = single(SampleTime_div_Ld*(d_phase_voltage_per_switching_state-id_k_1*Rs+omega_el*Lq*iq_k_1)+id_k_1);
        iq_k_2 = single(SampleTime_div_Lq*(q_phase_voltage_per_switching_state-iq_k_1*Rs-omega_el*(psiPM+id_k_1*Ld))+iq_k_1);
        ix_k_2 = single(SampleTime_div_Lx*(x_phase_voltage_per_switching_state-ix_k_1*Rs)+ix_k_1);
        iy_k_2 = single(SampleTime_div_Ly*(y_phase_voltage_per_switching_state-iy_k_1*Rs)+iy_k_1);
        
        % Calculation of the cost function
        J = single((id_ref-id_k_2)^2+(iq_ref-iq_k_2)^2+(ix_ref-ix_k_2)^2+(iy_ref-iy_k_2)^2);

end

== matlab function parallel_prediction_and_cost_function_6phase/Prediction_and_cost_function/Subsystem/MATLAB Function9 ==
  data: SampleTime_div_Ld input; J output; SampleTime_div_Lq input; SampleTime_div_Lx input; SampleTime_div_Ly input; id_k_1 input; iq_k_1 input; ix_k_1 input; iy_k_1 input; Rs input; omega_el input; Lq input; Ld input; psiPM input; d_phase_voltage_per_switching_state input; q_phase_voltage_per_switching_state input; x_phase_voltage_per_switching_state input; y_phase_voltage_per_switching_state input; id_ref input; iq_ref input; ix_ref input; iy_ref input
function J = fcn(SampleTime_div_Ld, SampleTime_div_Lq, SampleTime_div_Lx, SampleTime_div_Ly, id_k_1, iq_k_1, ix_k_1, iy_k_1, Rs, omega_el, Lq, Ld, psiPM, d_phase_voltage_per_switching_state, q_phase_voltage_per_switching_state, x_phase_voltage_per_switching_state, y_phase_voltage_per_switching_state, id_ref, iq_ref, ix_ref, iy_ref)
     
        % Prediction of the d-, q-, x-, y-currents of the 6-Phase-PMSM with the finite control set 
        id_k_2 = single(SampleTime_div_Ld*(d_phase_voltage_per_switching_state-id_k_1*Rs+omega_el*Lq*iq_k_1)+id_k_1);
        iq_k_2 = single(SampleTime_div_Lq*(q_phase_voltage_per_switching_state-iq_k_1*Rs-omega_el*(psiPM+id_k_1*Ld))+iq_k_1);
        ix_k_2 = single(SampleTime_div_Lx*(x_phase_voltage_per_switching_state-ix_k_1*Rs)+ix_k_1);
        iy_k_2 = single(SampleTime_div_Ly*(y_phase_voltage_per_switching_state-iy_k_1*Rs)+iy_k_1);
        
        % Calculation of the cost function
        J = single((id_ref-id_k_2)^2+(iq_ref-iq_k_2)^2+(ix_ref-ix_k_2)^2+(iy_ref-iy_k_2)^2);

end

== matlab function parallel_prediction_and_cost_function_6phase/Prediction_and_cost_function/Subsystem/MATLAB Function10 ==
  data: SampleTime_div_Ld input; J output; SampleTime_div_Lq input; SampleTime_div_Lx input; SampleTime_div_Ly input; id_k_1 input; iq_k_1 input; ix_k_1 input; iy_k_1 input; Rs input; omega_el input; Lq input; Ld input; psiPM input; d_phase_voltage_per_switching_state input; q_phase_voltage_per_switching_state input; x_phase_voltage_per_switching_state input; y_phase_voltage_per_switching_state input; id_ref input; iq_ref input; ix_ref input; iy_ref input
function J = fcn(SampleTime_div_Ld, SampleTime_div_Lq, SampleTime_div_Lx, SampleTime_div_Ly, id_k_1, iq_k_1, ix_k_1, iy_k_1, Rs, omega_el, Lq, Ld, psiPM, d_phase_voltage_per_switching_state, q_phase_voltage_per_switching_state, x_phase_voltage_per_switching_state, y_phase_voltage_per_switching_state, id_ref, iq_ref, ix_ref, iy_ref)
     
        % Prediction of the d-, q-, x-, y-currents of the 6-Phase-PMSM with the finite control set 
        id_k_2 = single(SampleTime_div_Ld*(d_phase_voltage_per_switching_state-id_k_1*Rs+omega_el*Lq*iq_k_1)+id_k_1);
        iq_k_2 = single(SampleTime_div_Lq*(q_phase_voltage_per_switching_state-iq_k_1*Rs-omega_el*(psiPM+id_k_1*Ld))+iq_k_1);
        ix_k_2 = single(SampleTime_div_Lx*(x_phase_voltage_per_switching_state-ix_k_1*Rs)+ix_k_1);
        iy_k_2 = single(SampleTime_div_Ly*(y_phase_voltage_per_switching_state-iy_k_1*Rs)+iy_k_1);
        
        % Calculation of the cost function
        J = single((id_ref-id_k_2)^2+(iq_ref-iq_k_2)^2+(ix_ref-ix_k_2)^2+(iy_ref-iy_k_2)^2);

end

== matlab function parallel_prediction_and_cost_function_6phase/Prediction_and_cost_function/Subsystem/MATLAB Function11 ==
  data: SampleTime_div_Ld input; J output; SampleTime_div_Lq input; SampleTime_div_Lx input; SampleTime_div_Ly input; id_k_1 input; iq_k_1 input; ix_k_1 input; iy_k_1 input; Rs input; omega_el input; Lq input; Ld input; psiPM input; d_phase_voltage_per_switching_state input; q_phase_voltage_per_switching_state input; x_phase_voltage_per_switching_state input; y_phase_voltage_per_switching_state input; id_ref input; iq_ref input; ix_ref input; iy_ref input
function J = fcn(SampleTime_div_Ld, SampleTime_div_Lq, SampleTime_div_Lx, SampleTime_div_Ly, id_k_1, iq_k_1, ix_k_1, iy_k_1, Rs, omega_el, Lq, Ld, psiPM, d_phase_voltage_per_switching_state, q_phase_voltage_per_switching_state, x_phase_voltage_per_switching_state, y_phase_voltage_per_switching_state, id_ref, iq_ref, ix_ref, iy_ref)
     
        % Prediction of the d-, q-, x-, y-currents of the 6-Phase-PMSM with the finite control set 
        id_k_2 = single(SampleTime_div_Ld*(d_phase_voltage_per_switching_state-id_k_1*Rs+omega_el*Lq*iq_k_1)+id_k_1);
        iq_k_2 = single(SampleTime_div_Lq*(q_phase_voltage_per_switching_state-iq_k_1*Rs-omega_el*(psiPM+id_k_1*Ld))+iq_k_1);
        ix_k_2 = single(SampleTime_div_Lx*(x_phase_voltage_per_switching_state-ix_k_1*Rs)+ix_k_1);
        iy_k_2 = single(SampleTime_div_Ly*(y_phase_voltage_per_switching_state-iy_k_1*Rs)+iy_k_1);
        
        % Calculation of the cost function
        J = single((id_ref-id_k_2)^2+(iq_ref-iq_k_2)^2+(ix_ref-ix_k_2)^2+(iy_ref-iy_k_2)^2);

end

== matlab function parallel_prediction_and_cost_function_6phase/Prediction_and_cost_function/Subsystem/MATLAB Function12 ==
  data: SampleTime_div_Ld input; J output; SampleTime_div_Lq input; SampleTime_div_Lx input; SampleTime_div_Ly input; id_k_1 input; iq_k_1 input; ix_k_1 input; iy_k_1 input; Rs input; omega_el input; Lq input; Ld input; psiPM input; d_phase_voltage_per_switching_state input; q_phase_voltage_per_switching_state input; x_phase_voltage_per_switching_state input; y_phase_voltage_per_switching_state input; id_ref input; iq_ref input; ix_ref input; iy_ref input
function J = fcn(SampleTime_div_Ld, SampleTime_div_Lq, SampleTime_div_Lx, SampleTime_div_Ly, id_k_1, iq_k_1, ix_k_1, iy_k_1, Rs, omega_el, Lq, Ld, psiPM, d_phase_voltage_per_switching_state, q_phase_voltage_per_switching_state, x_phase_voltage_per_switching_state, y_phase_voltage_per_switching_state, id_ref, iq_ref, ix_ref, iy_ref)
     
        % Prediction of the d-, q-, x-, y-currents of the 6-Phase-PMSM with the finite control set 
        id_k_2 = single(SampleTime_div_Ld*(d_phase_voltage_per_switching_state-id_k_1*Rs+omega_el*Lq*iq_k_1)+id_k_1);
        iq_k_2 = single(SampleTime_div_Lq*(q_phase_voltage_per_switching_state-iq_k_1*Rs-omega_el*(psiPM+id_k_1*Ld))+iq_k_1);
        ix_k_2 = single(SampleTime_div_Lx*(x_phase_voltage_per_switching_state-ix_k_1*Rs)+ix_k_1);
        iy_k_2 = single(SampleTime_div_Ly*(y_phase_voltage_per_switching_state-iy_k_1*Rs)+iy_k_1);
        
        % Calculation of the cost function
        J = single((id_ref-id_k_2)^2+(iq_ref-iq_k_2)^2+(ix_ref-ix_k_2)^2+(iy_ref-iy_k_2)^2);

end

== matlab function parallel_prediction_and_cost_function_6phase/Prediction_and_cost_function/Subsystem/MATLAB Function13 ==
  data: SampleTime_div_Ld input; J output; SampleTime_div_Lq input; SampleTime_div_Lx input; SampleTime_div_Ly input; id_k_1 input; iq_k_1 input; ix_k_1 input; iy_k_1 input; Rs input; omega_el input; Lq input; Ld input; psiPM input; d_phase_voltage_per_switching_state input; q_phase_voltage_per_switching_state input; x_phase_voltage_per_switching_state input; y_phase_voltage_per_switching_state input; id_ref input; iq_ref input; ix_ref input; iy_ref input
function J = fcn(SampleTime_div_Ld, SampleTime_div_Lq, SampleTime_div_Lx, SampleTime_div_Ly, id_k_1, iq_k_1, ix_k_1, iy_k_1, Rs, omega_el, Lq, Ld, psiPM, d_phase_voltage_per_switching_state, q_phase_voltage_per_switching_state, x_phase_voltage_per_switching_state, y_phase_voltage_per_switching_state, id_ref, iq_ref, ix_ref, iy_ref)
     
        % Prediction of the d-, q-, x-, y-currents of the 6-Phase-PMSM with the finite control set 
        id_k_2 = single(SampleTime_div_Ld*(d_phase_voltage_per_switching_state-id_k_1*Rs+omega_el*Lq*iq_k_1)+id_k_1);
        iq_k_2 = single(SampleTime_div_Lq*(q_phase_voltage_per_switching_state-iq_k_1*Rs-omega_el*(psiPM+id_k_1*Ld))+iq_k_1);
        ix_k_2 = single(SampleTime_div_Lx*(x_phase_voltage_per_switching_state-ix_k_1*Rs)+ix_k_1);
        iy_k_2 = single(SampleTime_div_Ly*(y_phase_voltage_per_switching_state-iy_k_1*Rs)+iy_k_1);
        
        % Calculation of the cost function
        J = single((id_ref-id_k_2)^2+(iq_ref-iq_k_2)^2+(ix_ref-ix_k_2)^2+(iy_ref-iy_k_2)^2);

end

== matlab function parallel_prediction_and_cost_function_6phase/Prediction_and_cost_function/Subsystem/MATLAB Function14 ==
  data: SampleTime_div_Ld input; J output; SampleTime_div_Lq input; SampleTime_div_Lx input; SampleTime_div_Ly input; id_k_1 input; iq_k_1 input; ix_k_1 input; iy_k_1 input; Rs input; omega_el input; Lq input; Ld input; psiPM input; d_phase_voltage_per_switching_state input; q_phase_voltage_per_switching_state input; x_phase_voltage_per_switching_state input; y_phase_voltage_per_switching_state input; id_ref input; iq_ref input; ix_ref input; iy_ref input
function J = fcn(SampleTime_div_Ld, SampleTime_div_Lq, SampleTime_div_Lx, SampleTime_div_Ly, id_k_1, iq_k_1, ix_k_1, iy_k_1, Rs, omega_el, Lq, Ld, psiPM, d_phase_voltage_per_switching_state, q_phase_voltage_per_switching_state, x_phase_voltage_per_switching_state, y_phase_voltage_per_switching_state, id_ref, iq_ref, ix_ref, iy_ref)
     
        % Prediction of the d-, q-, x-, y-currents of the 6-Phase-PMSM with the finite control set 
        id_k_2 = single(SampleTime_div_Ld*(d_phase_voltage_per_switching_state-id_k_1*Rs+omega_el*Lq*iq_k_1)+id_k_1);
        iq_k_2 = single(SampleTime_div_Lq*(q_phase_voltage_per_switching_state-iq_k_1*Rs-omega_el*(psiPM+id_k_1*Ld))+iq_k_1);
        ix_k_2 = single(SampleTime_div_Lx*(x_phase_voltage_per_switching_state-ix_k_1*Rs)+ix_k_1);
        iy_k_2 = single(SampleTime_div_Ly*(y_phase_voltage_per_switching_state-iy_k_1*Rs)+iy_k_1);
        
        % Calculation of the cost function
        J = single((id_ref-id_k_2)^2+(iq_ref-iq_k_2)^2+(ix_ref-ix_k_2)^2+(iy_ref-iy_k_2)^2);

end

== matlab function parallel_prediction_and_cost_function_6phase/Prediction_and_cost_function/Subsystem/MATLAB Function15 ==
  data: SampleTime_div_Ld input; J output; SampleTime_div_Lq input; SampleTime_div_Lx input; SampleTime_div_Ly input; id_k_1 input; iq_k_1 input; ix_k_1 input; iy_k_1 input; Rs input; omega_el input; Lq input; Ld input; psiPM input; d_phase_voltage_per_switching_state input; q_phase_voltage_per_switching_state input; x_phase_voltage_per_switching_state input; y_phase_voltage_per_switching_state input; id_ref input; iq_ref input; ix_ref input; iy_ref input
function J = fcn(SampleTime_div_Ld, SampleTime_div_Lq, SampleTime_div_Lx, SampleTime_div_Ly, id_k_1, iq_k_1, ix_k_1, iy_k_1, Rs, omega_el, Lq, Ld, psiPM, d_phase_voltage_per_switching_state, q_phase_voltage_per_switching_state, x_phase_voltage_per_switching_state, y_phase_voltage_per_switching_state, id_ref, iq_ref, ix_ref, iy_ref)
     
        % Prediction of the d-, q-, x-, y-currents of the 6-Phase-PMSM with the finite control set 
        id_k_2 = single(SampleTime_div_Ld*(d_phase_voltage_per_switching_state-id_k_1*Rs+omega_el*Lq*iq_k_1)+id_k_1);
        iq_k_2 = single(SampleTime_div_Lq*(q_phase_voltage_per_switching_state-iq_k_1*Rs-omega_el*(psiPM+id_k_1*Ld))+iq_k_1);
        ix_k_2 = single(SampleTime_div_Lx*(x_phase_voltage_per_switching_state-ix_k_1*Rs)+ix_k_1);
        iy_k_2 = single(SampleTime_div_Ly*(y_phase_voltage_per_switching_state-iy_k_1*Rs)+iy_k_1);
        
        % Calculation of the cost function
        J = single((id_ref-id_k_2)^2+(iq_ref-iq_k_2)^2+(ix_ref-ix_k_2)^2+(iy_ref-iy_k_2)^2);

end

== matlab function parallel_prediction_and_cost_function_6phase/Prediction_and_cost_function/Subsystem/MATLAB Function1 ==
  data: SampleTime_div_Ld input; J output; SampleTime_div_Lq input; SampleTime_div_Lx input; SampleTime_div_Ly input; id_k_1 input; iq_k_1 input; ix_k_1 input; iy_k_1 input; Rs input; omega_el input; Lq input; Ld input; psiPM input; d_phase_voltage_per_switching_state input; q_phase_voltage_per_switching_state input; x_phase_voltage_per_switching_state input; y_phase_voltage_per_switching_state input; id_ref input; iq_ref input; ix_ref input; iy_ref input
function J = fcn(SampleTime_div_Ld, SampleTime_div_Lq, SampleTime_div_Lx, SampleTime_div_Ly, id_k_1, iq_k_1, ix_k_1, iy_k_1, Rs, omega_el, Lq, Ld, psiPM, d_phase_voltage_per_switching_state, q_phase_voltage_per_switching_state, x_phase_voltage_per_switching_state, y_phase_voltage_per_switching_state, id_ref, iq_ref, ix_ref, iy_ref)
     
        % Prediction of the d-, q-, x-, y-currents of the 6-Phase-PMSM with the finite control set 
        id_k_2 = single(SampleTime_div_Ld*(d_phase_voltage_per_switching_state-id_k_1*Rs+omega_el*Lq*iq_k_1)+id_k_1);
        iq_k_2 = single(SampleTime_div_Lq*(q_phase_voltage_per_switching_state-iq_k_1*Rs-omega_el*(psiPM+id_k_1*Ld))+iq_k_1);
        ix_k_2 = single(SampleTime_div_Lx*(x_phase_voltage_per_switching_state-ix_k_1*Rs)+ix_k_1);
        iy_k_2 = single(SampleTime_div_Ly*(y_phase_voltage_per_switching_state-iy_k_1*Rs)+iy_k_1);
        
        % Calculation of the cost function
        J = single((id_ref-id_k_2)^2+(iq_ref-iq_k_2)^2+(ix_ref-ix_k_2)^2+(iy_ref-iy_k_2)^2);

end
